simulink model "Test_Decoder"  (Simulink 8.1)
settings: Solver=ode45  StartTime=0.0  StopTime=10.0  RelTol=1e-3
libraries: commutil2 x6, Computer_Library x3
settings Model: Creator=N  LastModifiedBy=uzivatel
settings DataIOCC: LimitDataPoints=off  SignalLoggingSaveFormat=Dataset
settings OptimizationCC: ExpressionDepthLimit=128
settings DebuggingCC: UnderspecifiedInitializationDetection=Simplified  MergeDetectMultiDrivingBlocksExec=error  SolverPrmCheckMsg=none  FcnCallInpInsideContextMsg=EnableAllAsError  FrameProcessingCompatibilityMsg=error  StateNameClashWarn=none
settings HardwareCC: ProdBitPerPointer=64  ProdLargestAtomicFloat=Float  ProdIntDivRoundTo=Zero  ProdEndianess=LittleEndian  ProdHWDeviceType=Intel->x86-64 (Windows64)
settings ModelReferenceCC: PropagateSignalLabelsOutOfModel=on
settings GRTTargetCC: CodeReplacementLibrary=None  CombineOutputUpdateFcns=on  CPPClassGenCompliant=on  GRTInterface=off

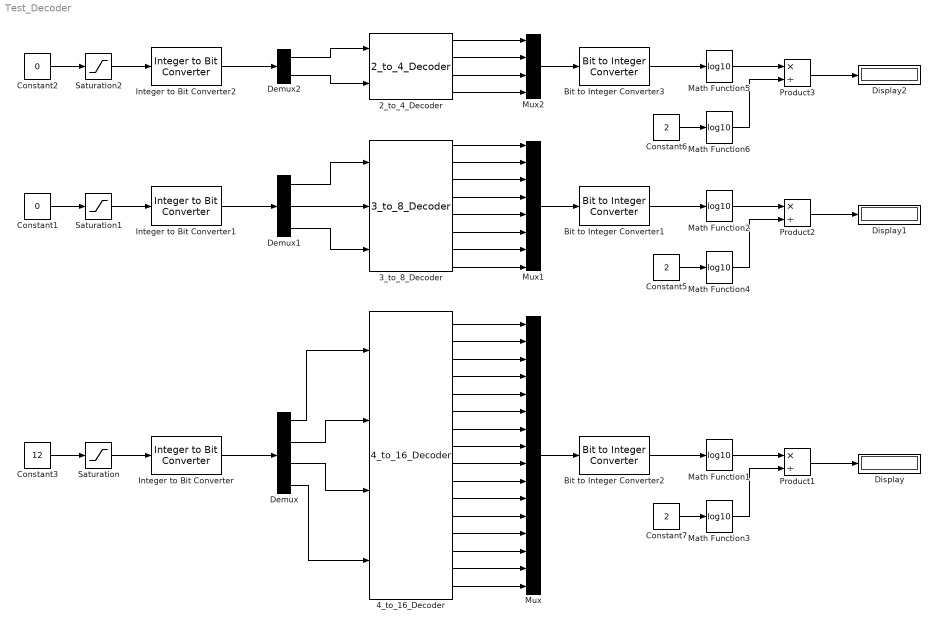
== system Test_Decoder ==
  2_to_4_Decoder : Computer_Library/Decoders/2_to_4_Decoder
  3_to_8_Decoder : Computer_Library/Decoders/3_to_8_Decoder
  4_to_16_Decoder : Computer_Library/Decoders/4_to_16_Decoder
  Bit to Integer Converter1 : commutil2/Bit to Integer Converter  nbits=8  bitOrder=LSB first  signedOutputValues=Unsigned  outDtype=single  outDtypeSigned=Inherit via internal rule
  Bit to Integer Converter2 : commutil2/Bit to Integer Converter  nbits=16  bitOrder=LSB first  signedOutputValues=Unsigned  outDtype=single  outDtypeSigned=Inherit via internal rule
  Bit to Integer Converter3 : commutil2/Bit to Integer Converter  nbits=4  bitOrder=LSB first  signedOutputValues=Unsigned  outDtype=single  outDtypeSigned=Inherit via internal rule
  Constant1 : Constant  Value=0  OutDataTypeStr=int16
  Constant2 : Constant  Value=0  OutDataTypeStr=int16
  Constant3 : Constant  Value=12  OutDataTypeStr=int16
  Constant5 : Constant  Value=2  OutDataTypeStr=single
  Constant6 : Constant  Value=2  OutDataTypeStr=single
  Constant7 : Constant  Value=2  OutDataTypeStr=single
  Demux : Demux
  Demux1 : Demux  Outputs=3
  Demux2 : Demux  Outputs=2
  Display : Display
  Display1 : Display
  Display2 : Display
  Integer to Bit Converter : commutil2/Integer to Bit Converter  nbits=4  signedInputValues=Unsigned  bitOrder=LSB first  outDtype=uint16
  Integer to Bit Converter1 : commutil2/Integer to Bit Converter  nbits=3  signedInputValues=Unsigned  bitOrder=LSB first  outDtype=uint16
  Integer to Bit Converter2 : commutil2/Integer to Bit Converter  nbits=2  signedInputValues=Unsigned  bitOrder=LSB first  outDtype=uint16
  Math Function1 : Math  Operator=log10  OutputSignalType=real  SaturateOnIntegerOverflow=on
  Math Function2 : Math  Operator=log10  OutputSignalType=real  SaturateOnIntegerOverflow=on
  Math Function3 : Math  Operator=log10  SaturateOnIntegerOverflow=on
  Math Function4 : Math  Operator=log10  SaturateOnIntegerOverflow=on
  Math Function5 : Math  Operator=log10  OutputSignalType=real  SaturateOnIntegerOverflow=on
  Math Function6 : Math  Operator=log10  SaturateOnIntegerOverflow=on
  Mux : Mux  Inputs=16
  Mux1 : Mux  Inputs=8
  Mux2 : Mux
  Product1 : Product  Inputs=*/
  Product2 : Product  Inputs=*/
  Product3 : Product  Inputs=*/
  Saturation : Saturate  UpperLimit=15  LowerLimit=0
  Saturation1 : Saturate  UpperLimit=7  LowerLimit=0
  Saturation2 : Saturate  UpperLimit=3  LowerLimit=0
  wires:
  4_to_16_Decoder/1 -> Mux/1
  4_to_16_Decoder/2 -> Mux/2
  4_to_16_Decoder/3 -> Mux/3
  4_to_16_Decoder/4 -> Mux/4
  4_to_16_Decoder/5 -> Mux/5
  4_to_16_Decoder/6 -> Mux/6
  4_to_16_Decoder/7 -> Mux/7
  4_to_16_Decoder/8 -> Mux/8
  4_to_16_Decoder/9 -> Mux/9
  4_to_16_Decoder/10 -> Mux/10
  4_to_16_Decoder/11 -> Mux/11
  4_to_16_Decoder/12 -> Mux/12
  4_to_16_Decoder/13 -> Mux/13
  4_to_16_Decoder/14 -> Mux/14
  4_to_16_Decoder/15 -> Mux/15
  4_to_16_Decoder/16 -> Mux/16
  Demux/1 -> 4_to_16_Decoder/1
  Demux/2 -> 4_to_16_Decoder/2
  Demux/3 -> 4_to_16_Decoder/3
  Demux/4 -> 4_to_16_Decoder/4
  Integer to Bit Converter/1 -> Demux/1
  Saturation/1 -> Integer to Bit Converter/1
  Constant3/1 -> Saturation/1
  3_to_8_Decoder/1 -> Mux1/1
  3_to_8_Decoder/8 -> Mux1/8
  3_to_8_Decoder/7 -> Mux1/7
  3_to_8_Decoder/6 -> Mux1/6
  3_to_8_Decoder/5 -> Mux1/5
  3_to_8_Decoder/4 -> Mux1/4
  3_to_8_Decoder/3 -> Mux1/3
  3_to_8_Decoder/2 -> Mux1/2
  2_to_4_Decoder/4 -> Mux2/4
  2_to_4_Decoder/3 -> Mux2/3
  2_to_4_Decoder/2 -> Mux2/2
  2_to_4_Decoder/1 -> Mux2/1
  Mux1/1 -> Bit to Integer Converter1/1
  Demux1/2 -> 3_to_8_Decoder/2
  Demux1/3 -> 3_to_8_Decoder/3
  Demux1/1 -> 3_to_8_Decoder/1
  Demux2/1 -> 2_to_4_Decoder/1
  Demux2/2 -> 2_to_4_Decoder/2
  Integer to Bit Converter1/1 -> Demux1/1
  Integer to Bit Converter2/1 -> Demux2/1
  Saturation1/1 -> Integer to Bit Converter1/1
  Saturation2/1 -> Integer to Bit Converter2/1
  Constant1/1 -> Saturation1/1
  Constant2/1 -> Saturation2/1
  Mux/1 -> Bit to Integer Converter2/1
  Bit to Integer Converter2/1 -> Math Function1/1
  Math Function1/1 -> Product1/1
  Product1/1 -> Display/1
  Constant7/1 -> Math Function3/1
  Math Function3/1 -> Product1/2
  Bit to Integer Converter1/1 -> Math Function2/1
  Math Function2/1 -> Product2/1
  Product2/1 -> Display1/1
  Constant5/1 -> Math Function4/1
  Math Function4/1 -> Product2/2
  Bit to Integer Converter3/1 -> Math Function5/1
  Math Function5/1 -> Product3/1
  Product3/1 -> Display2/1
  Constant6/1 -> Math Function6/1
  Math Function6/1 -> Product3/2
  Mux2/1 -> Bit to Integer Converter3/1
